simulink model "fausto_model"  (R2024b)
settings: Solver=VariableStepAuto  StartTime=0.0  StopTime=10.0  RelTol=1e-3
model workspace (MAT data in the model file):
  Dm = Simulink.Parameter
  Dm.Complexity = 'real'
  Dm.Dimensions = [0 0]
  Dm.DataType = 'auto'
values from neighbouring files (symbols this model uses):
  beta = 1    [init_params.m]
  C = 1    [init_params.m]
  Cr = 1    [init_params.m]
  Dm = 0.00240    (= 0.0024)    [init_params.m]
  Dt = 0.167    [init_params.m]
  g = 9.81    [init_params.m]
  gamma = 0    [init_params.m]
  Jeq = Jr + Jh + Jprop    (= 4.40304e-05)    [init_params.m]
  Jp = 1    [init_params.m]
  Jr = 4.00e-6    (= 4e-06)    [init_params.m]
  Jyaw = 1    [init_params.m]
  Jz = 1    [init_params.m]
  ke = kt    (= 0.042)    [init_params.m]
  kt = 4.20e-2    (= 0.042)    [init_params.m]
  Md = 1.07    [init_params.m]
  Rm = 8.40    (= 8.4)    [init_params.m]
settings Model: Creator=donadi  LastModifiedBy=donadi

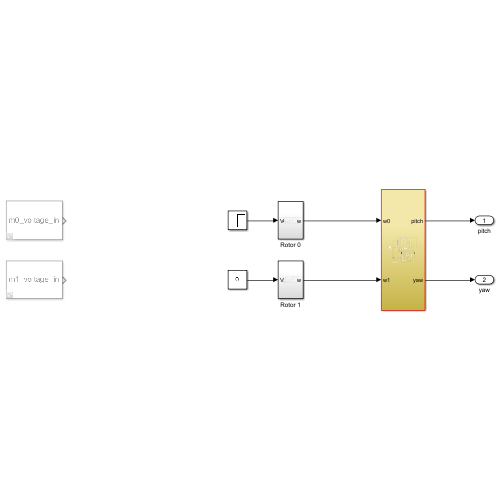
[thumbnail: Simulink's stored preview of the top-level diagram]
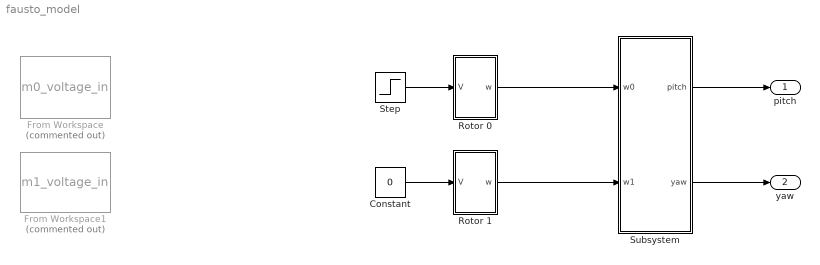
== system fausto_model ==
  Constant : Constant  Value=0
  From Workspace : FromWorkspace  Commented=on  VariableName=m0_voltage_in
  From Workspace1 : FromWorkspace  Commented=on  VariableName=m1_voltage_in
  Rotor 0 : Subsystem
  Rotor 1 : Subsystem
  Step : Step  SampleTime=0
  Subsystem : Subsystem
  pitch : Outport
  yaw : Outport  Port=2
  wires:
  Rotor 0/1(w) -> Subsystem/1(w0)
  Rotor 1/1(w) -> Subsystem/2(w1)
  Subsystem/1(pitch) -> pitch/1
  Subsystem/2(yaw) -> yaw/1
  Step/1 -> Rotor 0/1(V)
  Constant/1 -> Rotor 1/1(V)

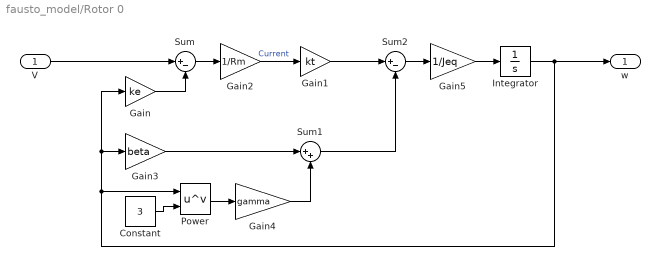
== system fausto_model/Rotor 0 ==
  V : Inport
  Constant : Constant  Value=3
  Gain : Gain  Gain=ke
  Gain1 : Gain  Gain=kt
  Gain2 : Gain  Gain=1/Rm
  Gain3 : Gain  Gain=beta
  Gain4 : Gain  Gain=gamma
  Gain5 : Gain  Gain=1/Jeq
  Integrator : Integrator
  Power : Math  Operator=pow
  Sum : Sum  Inputs=|+-
  Sum1 : Sum  Inputs=|++
  Sum2 : Sum  Inputs=|+-
  w : Outport
  wires:
  Gain3/1 -> Sum1/1
  V/1 -> Sum/1
  Gain1/1 -> Sum2/1
  Power/1 -> Gain4/1
  Gain2/1 -> Gain1/1  "Current"
  Gain/1 -> Sum/2
  Gain5/1 -> Integrator/1
  Sum1/1 -> Sum2/2
  Integrator/1 -> w/1, Power/1, Gain/1, Gain3/1
  Gain4/1 -> Sum1/2
  Sum/1 -> Gain2/1
  Sum2/1 -> Gain5/1
  Constant/1 -> Power/2

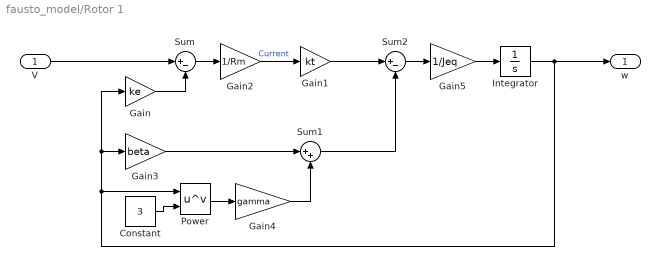
== system fausto_model/Rotor 1 ==
  V : Inport
  Constant : Constant  Value=3
  Gain : Gain  Gain=ke
  Gain1 : Gain  Gain=kt
  Gain2 : Gain  Gain=1/Rm
  Gain3 : Gain  Gain=beta
  Gain4 : Gain  Gain=gamma
  Gain5 : Gain  Gain=1/Jeq
  Integrator : Integrator
  Power : Math  Operator=pow
  Sum : Sum  Inputs=|+-
  Sum1 : Sum  Inputs=|++
  Sum2 : Sum  Inputs=|+-
  w : Outport
  wires:
  Gain3/1 -> Sum1/1
  V/1 -> Sum/1
  Gain1/1 -> Sum2/1
  Power/1 -> Gain4/1
  Gain2/1 -> Gain1/1  "Current"
  Gain/1 -> Sum/2
  Gain5/1 -> Integrator/1
  Sum1/1 -> Sum2/2
  Integrator/1 -> w/1, Power/1, Gain/1, Gain3/1
  Gain4/1 -> Sum1/2
  Sum/1 -> Gain2/1
  Sum2/1 -> Gain5/1
  Constant/1 -> Power/2

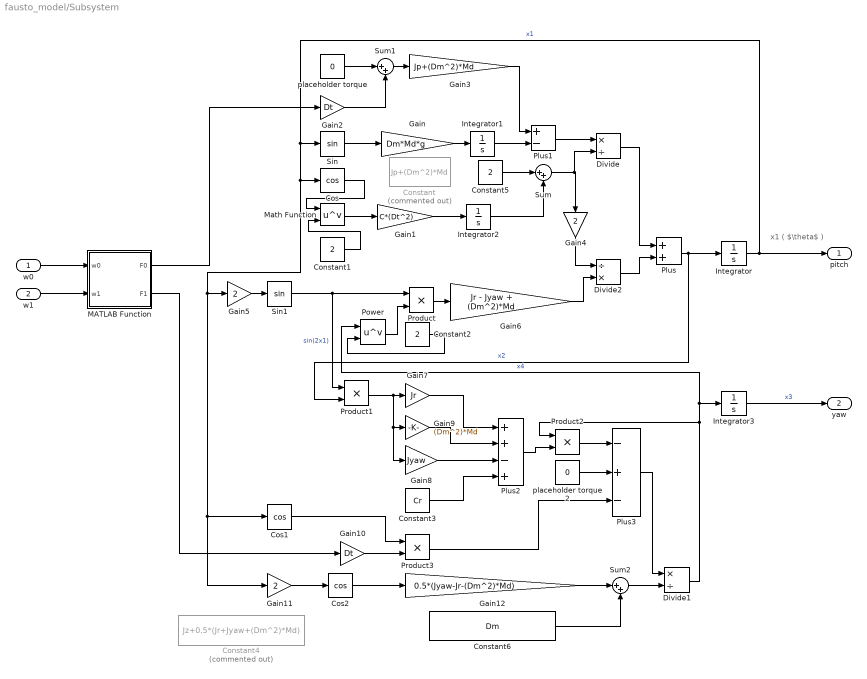
== system fausto_model/Subsystem ==
  note: x1 ( $\theta$ )
  w0 : Inport
  w1 : Inport  Port=2
  Constant : Constant  Commented=on  Value=Jp+(Dm^2)*Md
  Constant1 : Constant  Value=2
  Constant2 : Constant  Value=2
  Constant3 : Constant  Value=Cr
  Constant4 : Constant  Commented=on  Value=Jz+0.5*(Jr+Jyaw+(Dm^2)*Md)
  Constant5 : Constant  Value=2
  Constant6 : Constant  Value=Dm
  Cos : Trigonometry  Operator=cos
  Cos1 : Trigonometry  Operator=cos
  Cos2 : Trigonometry  Operator=cos
  Divide : Product  Inputs=*/
  Divide1 : Product  Inputs=*/
  Divide2 : Product  Inputs=/*
  Gain : Gain  Gain=Dm*Md*g
  Gain1 : Gain  Gain=C*(Dt^2)
  Gain10 : Gain  Gain=Dt
  Gain11 : Gain  Gain=2
  Gain12 : Gain  Gain=0.5*(Jyaw-Jr-(Dm^2)*Md)
  Gain2 : Gain  Gain=Dt
  Gain3 : Gain  Gain=Jp+(Dm^2)*Md
  Gain4 : Gain  Gain=2
  Gain5 : Gain  Gain=2
  Gain6 : Gain  Gain=Jr - Jyaw + (Dm^2)*Md
  Gain7 : Gain  Gain=Jr
  Gain8 : Gain  Gain=Jyaw
  Gain9 : Gain  Gain=(Dm^2)*Md
  Integrator{,1..3} (4 alike) : Integrator
  MATLAB Function : MATLAB Function  TreatAsAtomicUnit=on
  Math Function : Math  Operator=pow
  Plus : Sum
  Plus1 : Sum  Inputs=+-
  Plus2 : Sum  Inputs=++-+
  Plus3 : Sum  Inputs=-+-
  Power : Math  Operator=pow
  Product{,1..3} (4 alike) : Product
  Sin : Trigonometry
  Sin1 : Trigonometry
  Sum : Sum  Inputs=|++
  Sum1 : Sum  Inputs=|++
  Sum2 : Sum  Inputs=|++
  placeholder torque : Constant  Value=0
  placeholder torque 2 : Constant  Value=0
  pitch : Outport
  yaw : Outport  Port=2
  wires:
  Divide/1 -> Plus/1
  Constant1/1 -> Math Function/2
  placeholder torque 2/1 -> Plus3/2
  Integrator1/1 -> Plus1/2
  Gain10/1 -> Product3/2
  Product/1 -> Gain6/1
  Plus3/1 -> Divide1/1
  Divide1/1 -> Integrator3/1, Power/1, Product2/1  "x4"
  Plus2/1 -> Product2/2
  Plus1/1 -> Divide/1
  Divide2/1 -> Plus/2
  Power/1 -> Product/2
  Math Function/1 -> Gain1/1
  w1/1 -> MATLAB Function/2(w1)
  Gain2/1 -> Sum1/2
  Constant3/1 -> Plus2/4
  Integrator3/1 -> yaw/1  "x3"
  Product1/1 -> Gain9/1, Gain8/1, Gain7/1
  Gain9/1 -> Plus2/2
  Gain11/1 -> Cos2/1
  Integrator/1 -> pitch/1, Gain11/1, Cos1/1, Gain5/1, Cos/1, Sin/1  "x1"
  Product3/1 -> Plus3/3
  Sum/1 -> Gain4/1, Divide/2
  Plus/1 -> Product1/2, Integrator/1  "x2"
  Constant2/1 -> Power/2
  Gain6/1 -> Divide2/2
  Sin1/1 -> Product1/1, Product/1  "sin(2x1)"
  Sin/1 -> Gain/1
  MATLAB Function/1(F0) -> Gain2/1
  Cos/1 -> Math Function/1
  Gain8/1 -> Plus2/3
  Gain5/1 -> Sin1/1
  Product2/1 -> Plus3/1
  Gain4/1 -> Divide2/1
  Gain/1 -> Integrator1/1
  Sum1/1 -> Gain3/1
  Gain3/1 -> Plus1/1
  Cos2/1 -> Gain12/1
  placeholder torque/1 -> Sum1/1
  MATLAB Function/2(F1) -> Gain10/1
  Sum2/1 -> Divide1/2
  w0/1 -> MATLAB Function/1(w0)
  Gain1/1 -> Integrator2/1
  Cos1/1 -> Product3/1
  Gain12/1 -> Sum2/1
  Integrator2/1 -> Sum/2
  Gain7/1 -> Plus2/1
  Constant5/1 -> Sum/1
  Constant6/1 -> Sum2/2

== matlab function fausto_model/Subsystem/MATLAB Function ==
  data: w0 input; F0 output; w1 input; F1 output
function [F0,F1] = fcn(w0, w1)
if w0>=0
    F0 = k0pp1*w0^2 + k0pp2*w0;
else
    F0 = k0pn1*w0^2 + k0pn2*w0;
end
if w1>=0
    F1 = k1pp1*w1^2 + k1pp2*w1;
else
    F1 = k1pn1*w1^2 + k1pn2*w1;
end
